simulink model "VCMGCM1962020b_v2"  (R2020b)
settings: Solver=FixedStepDiscrete  StartTime=0.0  StopTime=10.0  FixedStep=0.005  RelTol=1e-3  EnableMultiTasking=on
PreLoadFcn:
  | try, model_open; catch, disp('Error occurred while executing model pre-load callback: model_open.m'); disp('Please assure that the MATLAB working directory is set to the model directory before opening.'); end
InitFcn:
  | try, model_open; catch, end
undefined symbols (not defined in the file): Bridge, GCM, H, raptor_get_param_eval, raptor_get_safe_string, raptor_xcp_function
libraries: Blocks_lib x1165, Raptor_lib x665, simulink x62, VCM_lib x5
(part 1 of 23)
CloseFcn:
  | try, model_close; catch, end
settings Model: MotoHawkBuildVersion=501  MotoHawkBuildStats=struct('TotalFLASH',{0},'TotalEEPROM',{0},'TotalRAM',{0},'AppFLASH',{0},'AppEEPROM',{0},'AppRAM',{0},'HeapRAM',{0},'BuildSuccessCount',{170},'BuildErrorCount',{28})  MotoHawkModelSavedName=EVCM  MotoHawkModelGUID=11a0a5ad-fc23-4ada-98-f8-de-ae-e5-cd-40  MotoHawkModelOpenTime=2015 6 17 13 8 21.706  MotoHawkModelElapsedTime=81984019.981  MotoHawkBuildInfo=struct('model_name',{'EVCM'},'motohawk_version',{'2013a_sp0.336'},'motohawk_component_version',{'0.0.8'},'matlab_version',{'7.14.0'},'build_version',{'500'},'module_type',{'ECM-5554-112-0904-xD'},'layout_type',{'DEV'},'processor_family',{'MotoCoder'},'processor_type',{'MPC5554'},'toolchain_vendor',{'gcc-powerpc-eabispe'},'toolchain_version',{'4.6.0'},'component',{logical(0)},'archive_file',{''},'enable_build',{1},'fptype',{0},'flash_size',{2097152},'ee_size',{0},'ram_size',{65536},'decram_size',{0},'eri_table0_rev',{9},'max_eri_table_size',{65535},'use_debug_vardecs',{1},'use_info_vardecs',{1},'fgnd_base_period_ms',{5},'bgnd_base_period_ms',{100},'build_dir',{'C:\Users\Joe Morbitzer\Documents\Work - New Eagle\Projects\Base EV Supervisor Kit\EVCM_New\EVCM_Build'},'dll_name',{'EVCM_500'},'srz_name',{'EVCM_500'},'fgnd_stack_size',{3072},'fgnd_angle_stack_size',{0},'bgnd_stack_size',{2048},'idle_stack_size',{2048},'irq_stack_size',{1536},'heap_size',{4096},'heap_margin',{409},'install_dll_dir',{'C:\ECUFiles\TDBDLL'},'install_srz_dir',{'C:\ECUFiles\Programs\'},'app_int_stack_size',{2048},'shutdown_stack_size',{2048},'mingw_dir',{'C:\Program Files (x86)\Woodward\DevelopmentTools\Toolchains\GCC\win32-pe\4_4_0\'},'motohawk_dir',{'C:\Program Files (x86)\Woodward\MCS\MotoHawk\2013a_sp0.336'},'toolchain_dir',{'C:\Program Files (x86)\Woodward\DevelopmentTools\Toolchains\GCC\powerpc-eabispe\4_6_0'},'matlab_root',{'C:\Program Files\MATLAB\R2012a'},'model_guid',{'11a0a5ad-fc23-4ada-98-f8-de-ae-e5-cd-40'},'build_guid',{'47747e62-59be-442a-8d-e0-87-3b-e1-68-f2'},'token_guid',{'24876F82C12F5B448488EC225C14CAFD'})  MotoHawkBuildGUID=47747e62-59be-442a-8d-e0-87-3b-e1-68-f2  RegisteredStructs=struct('Name',{'FreezeFrame'},'Data',{struct('FltName',{0},'FltID',{0},'FltCount',{0},'RunTime',{0},'KeySw',{0})},'Enums',{{{'None','APP1InptHi','APP1InptLo','APP2InptHi','APP2InptLo','APPSnsCnflct','BPP1InptHi','BPP1InptLo','BPP2InptHi','BPP2InptLo','BPPSnsCnflct','DRVPVltHi','DRVPVltInptHi','DRVPVltInptLo','DRVPVltLo','EMTrqXChk','HVBCntrStck','HVBCurHi','HVBFlt','HVBNoTrnOn','HVBSOCLo','HVBTmpAvgHi1','HVBTmpAvgHi2','HVBTmpAvgHi3','HVBTmpAvgHi4','HVBTmpMxHi','HVBVltMnLo','HVBVltMxHi','HVSysFlt','KeySwVltHi','KeySwVltInptHi','KeySwVltInptLo','KeySwVltLo','MsgName1RxRateLo','MsgName2RxRateLo','PIMFlt','PIMNoTrnOn','PIMTmpHi1','PIMTmpHi2','PIMTmpHi3','PIMTmpHi4','Var11Inpt','Var21Inpt','VehSpdHi','XDRPVltHi','XDRPVltInptHi','XDRPVltInptLo','XDRPVltLo'},'',''}})  MotoHawkBuildDirectory=C:\Users\Joe Morbitzer\Documents\Work - New Eagle\Projects\Base EV Supervisor Kit\EVCM_New\EVCM_Build  RaptorUIDSize=4  Raptor_Target=GCM-1793-196-1503  Raptor_Calloc=NonVolatile (EEPROM)  RaptorFaultManager=OBD  RaptorBuildNum=67  Raptor_ecuaddr=253  Raptor_IsLiteMode=0  RaptorFaultManagerAddXYCounts=0  Creator=Joseph M. Morbitzer  LastModifiedBy=hratnam
settings ConfigSet: Description="This Simulink Configuration Set is preconfigured  for the MotoHawk target \"ECM-5554-112-0904-xD\"."
settings DataIOCC: LimitDataPoints=on  SaveFormat=Array  SignalLoggingSaveFormat=ModelDataLogs  ReturnWorkspaceOutputs=off
settings OptimizationCC: DefaultParameterBehavior=Inlined  UseSpecifiedMinMax=on  InlineInvariantSignals=on  EnhancedBackFolding=on  ExpressionDepthLimit=2147483647  InitFltsAndDblsToZero=on  NoFixptDivByZeroProtection=on  EfficientFloat2IntCast=on  LifeSpan=1  EfficientTunableParamExpr=on
settings DebuggingCC: ArtificialAlgebraicLoopMsg=none  InheritedTsInSrcMsg=none  TasksWithSamePriorityMsg=none  AllowSymbolicDim=off  StateNameClashWarn=warning  SFUnexpectedBacktrackingDiag=warning  SFNoUnconditionalDefaultTransitionDiag=warning  SFExecutionAtInitializationDiag=none  ArithmeticOperatorsInVariantConditions=warning
settings HardwareCC: ProdBitPerPointer=32  ProdBitPerSizeT=32  ProdBitPerPtrDiffT=32  ProdLargestAtomicFloat=None  ProdIntDivRoundTo=Undefined  ProdWordSize=32  ProdHWDeviceType=Infineon->TriCore  TargetIntDivRoundTo=Zero  TargetEndianess=LittleEndian  ProdEqTarget=off
settings ModelReferenceCC: UpdateModelReferenceTargets=AssumeUpToDate  CheckModelReferenceTargetMessage=none  ModelReferenceNumInstancesAllowed=Zero  PropagateSignalLabelsOutOfModel=off
settings SFSimCC: SimUseLocalCustomCode=off  MATLABDynamicMemAlloc=off  CustomCodeUndefinedFunction=UseInterfaceOnly
settings RTWCC: Description=Raptor (tm)  SystemTargetFile=raptor.tlc  GenCodeOnly=on  MakeCommand=raptor_make_rtw  TemplateMakefile=raptor.tmf  RTWUseLocalCustomCode=off
settings CodeAppCC: IgnoreCustomStorageClasses=off  MaxIdLength=100  CustomSymbolStrType=$N$R$M  CustomSymbolStrField=$H$N$M  StateflowObjectComments=on  InternalIdentifier=Classic
settings STFCustomTargetCC: GenerateSampleERTMain=on  ModelReferenceCompliant=off  ConcurrentExecutionCompliant=off  CombineOutputUpdateFcns=on  CombineSignalStateStructs=on  ERTCustomFileBanners=on  SupportComplex=off  SupportContinuousTime=off  SupportNonInlinedSFcns=off  RemoveResetFunc=on  MATLABClassNameForMDSCustomization=Simulink.SoftwareTarget.ERTCustomization  CPPClassGenCompliant=off  GRTInterface=off  SystemTargetFile=raptor.tlc
settings ERTTargetCC: MultiwordLength=2048  GenerateSampleERTMain=on  ModelReferenceCompliant=off  ParMdlRefBuildCompliant=off  CompOptLevelCompliant=off  ConcurrentExecutionCompliant=off  CombineSignalStateStructs=on  SupportComplex=off  ModelStepFunctionPrototypeControlCompliant=off  CPPClassGenCompliant=off  UseToolchainInfoCompliant=off  InlinedParameterPlacement=NonHierarchical  ERTCustomFileTemplate=example_file_process.tlc  SuppressUnreachableDefaultCases=off
settings ConfigComp: CovMetricSettings=dw  CovSaveCumulativeToWorkspaceVar=on  CovSaveSingleToWorkspaceVar=on  CovExternalEMLEnable=off

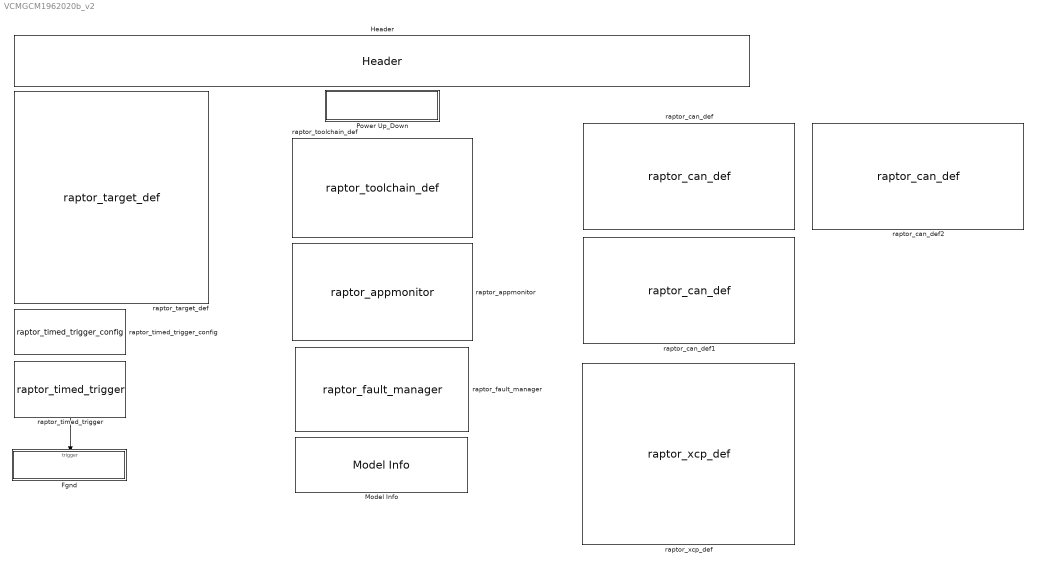
== system VCMGCM1962020b_v2 ==
  Fgnd : Subsystem  TreatAsAtomicUnit=on  mask{samptime=0.005}
      mask prompts: samptime "Sample Time (sec)"
      settings: RTWFcnNameOpts=Use subsystem name  RTWFileNameOpts=Use function name
      mask Display: disp(['Sample Time\n' num2str(samptime) ' sec']);
  Header : Blocks_lib/Header  width=Portrait  addtext=''
  Model Info : simulink/Model-Wide Utilities/Model Info  Frame=on  DisplayStringWithTags=|  HorizontalTextAlignment=Center  LeftAlignmentValue=0.5
      | Model Info
      | 
      | %<ModelVersion>
      | %<Description>
      | %<LastModifiedBy>
      | %<ModifiedComment>
  Power Up_Down : Subsystem  mask{group='Sensors | Voltage'}
  raptor_appmonitor : Raptor_lib/Application Monitoring/raptor_appmonitor  enabled=on  startupAction=Run  addStartupActionCal=off  minIdle=10  maxThread=70  calAccess=1  pctOverrunLimit=20  overrunAction=Count Occurrences  pauseOnReset=on  maxStackUsage=90  stackOverrunAction=Stop Application  addMaxStackCal=off  CANen=off
      settings: SourceProductName=Raptor
  raptor_can_def : Raptor_lib/CAN/raptor_can_def  canBus='CAN1'  resourceValues=CAN1|CAN2|CAN3|(None)  resource=CAN1  baudRateValues=125k|250k|500k|1000k  baudRate=250k  enable_baud_rate_config='RAPTOR MASK DEFAULT'  sim_func_name='RAPTOR MASK DEFAULT'  createButton=[]  txQueueSize=128  rxQueueSize=32
      settings: SourceProductName=Raptor
  raptor_can_def1 : Raptor_lib/CAN/raptor_can_def  canBus='CAN3'  resourceValues=CAN1|CAN2|CAN3|(None)  resource=CAN3  baudRateValues=125k|250k|500k|1000k  baudRate=500k  enable_baud_rate_config='RAPTOR MASK DEFAULT'  sim_func_name='RAPTOR MASK DEFAULT'  createButton=[]  txQueueSize=128  rxQueueSize=32
      settings: SourceProductName=Raptor
  raptor_can_def2 : Raptor_lib/CAN/raptor_can_def  canBus='CAN2'  resourceValues=CAN1|CAN2|CAN3|(None)  resource=CAN2  baudRateValues=125k|250k|500k|1000k  baudRate=250k  enable_baud_rate_config='RAPTOR MASK DEFAULT'  sim_func_name='RAPTOR MASK DEFAULT'  createButton=[]  txQueueSize=128  rxQueueSize=32
      settings: SourceProductName=Raptor
  raptor_fault_manager : Raptor_lib/Faults/raptor_fault_manager  button=0  managerTypeValues=Standard|OBD  managerType=OBD  cyclesToHeal=3  cyclesToClear=40  addXYCounts=0  calFaultMap=1  minFaultActions=2  minFaultTriggers=4  calAccessValues=4|3|2|1  calAccess=1  calFunction='Diagnostics'  initMap=struct()
      settings: SourceProductName=Raptor
  raptor_target_def : Raptor_lib/Configuration/raptor_target_def  targetValues=BCM-5646-48-1404|DISP-VC128-1901|DISP-VC320L-1402|DISP-VC320-1204|DISP-VC500-1904|DISP-VC700-2003|DISP-VC300R-2004|GCM-5634M-070-1459|GCM-5634M-070-1559|GCM-5634M-070-1562|ECM-1793-196-1503|GCM-1793-196-1503|GCM-5605B-048-1906|GCM-5607B-80-1901|GCM-5607B-80-1903|GCM-5607B-80-2001|RCM-5743R-080-2005|UAS-5743R-050-2006|GCM-5746R-048-1902|HCM-5604-36-1303|HCM-5604-36-1702  target=GCM-1793-196-1503  simpack=0  simulator=0  heap=2*1024  stack=2*1024  fgndStack=2*1024  bgndStack=2*1024  idleStack=1024  intStack=1536  sdStack=1024  appStack=1024  ecuaddr=253  uds_server_addr_ext=0  uds_server_addr=hex2dec('600')  uds_client_addr=hex2dec('650')  callocValues=Constant (FLASH)|NonVolatile (EEPROM)  calloc=NonVolatile (EEPROM)  compilerValues=HighTec v3.4.5.11  compiler=HighTec v3.4.5.11  setFileName=0  exeName=[raptor_get_safe_string(bdroot) '_']  addBuildNum=1  minVerChars=3  extraOutput=0  buildLocationValues=Raptor Default|Model Directory|User Defined  buildLocation=Raptor Default  exeLocation=''  a2lLocation=''  rpgLocation=''
      settings: SourceProductName=Raptor
  raptor_timed_trigger : Raptor_lib/Triggers/raptor_timed_trigger  triggerValues=Foreground|Foregroundx2|Foregroundx5|Foregroundx10|Foregroundx20|Background|Backgroundx2|Backgroundx5|Backgroundx10|Backgroundx20|Second|Minute  trigger=Foreground  inherited=0  alwaysEnabled=0  triggerPriority=0  triggerName=FGND_igkUo
      settings: SourceProductName=Raptor
  raptor_timed_trigger_config : Raptor_lib/Triggers/raptor_timed_trigger_config  triggerValues=Foreground|Background|Second|Minute  trigger=Foreground  period=5  CM2115newPeriod=5
      settings: SourceProductName=Raptor
  raptor_toolchain_def : Raptor_lib/Configuration/raptor_toolchain_def  matlabVer=9.9 (2020b)  raptorVer=2020b_2.2.13891  matCondition=Match Exactly  rapCondition=Match Exactly  matlabVerValues=9.9 (2020b)|9.8 (2020a)|9.7 (2019b)|9.6 (2019a)|9.5 (2018b)  matConditionValues=Match Exactly|Match or Newer|Match or Older  rapConditionValues=Match Exactly|Match or Newer|Match or Older
      settings: SourceProductName=Raptor
  raptor_xcp_def : Raptor_lib/Configuration/raptor_xcp_def  canBus='CAN1'  bcID=hex2dec('100')  bcID_TypeValues=Standard|Extended  bcID_Type=Standard  rxID=hex2dec('200')  rxID_TypeValues=Standard|Extended  rxID_Type=Standard  txID=hex2dec('300')  txID_TypeValues=Standard|Extended  txID_Type=Standard  daqRates=[5 10 100]  numODTs=80  genCANAPE=0  genVISION=0  securityValues=Standard|None|Custom User Defined  security=Standard  dllName=raptor_XCPSecurity.dll  accessValues=4|3|2|1  access=1
      settings: SourceProductName=Raptor
  wires:
  raptor_timed_trigger/1 -> Fgnd/Trigger

== system VCMGCM1962020b_v2/Fgnd ==
  f : TriggerPort  TriggerType=function-call  VariantControl=(inherit)
  Actuators : Subsystem
  Bus Creator : BusCreator  Inputs=5
  Bus Manager : Subsystem
  Control : Subsystem
  Diagnostics : Subsystem
  Header : Blocks_lib/Header  width=Portrait  addtext=''
  Sensors : Subsystem
  Virtual Sensors : Subsystem
  wires:
  Bus Manager/1(SBus) -> Sensors/1(Data)
  Bus Manager/2(VSBus) -> Virtual Sensors/1(Data)
  Bus Manager/3(CBus) -> Control/1(Data)
  Bus Manager/4(ABus) -> Actuators/1(Data)
  Bus Manager/5(DBus) -> Diagnostics/1(Data)
  Sensors/1(" Data") -> Bus Creator/1
  Virtual Sensors/1(" Data") -> Bus Creator/2
  Control/1(" Data") -> Bus Creator/3
  Actuators/1(" Data") -> Bus Creator/4
  Diagnostics/1(" Data") -> Bus Creator/5
  Bus Creator/1 -> Bus Manager/1(Data)

== system VCMGCM1962020b_v2/Power Up_Down ==
  Background : Subsystem
  raptor_timed_trigger : Raptor_lib/Triggers/raptor_timed_trigger  triggerValues=Foreground|Foregroundx2|Foregroundx5|Foregroundx10|Foregroundx20|Background|Backgroundx2|Backgroundx5|Backgroundx10|Backgroundx20|Second|Minute  trigger=Background  inherited=0  alwaysEnabled=1  triggerPriority=50  triggerName=BGND_kDJL0
      settings: SourceProductName=Raptor
  wires:
  raptor_timed_trigger/1 -> Background/Trigger

== system VCMGCM1962020b_v2/Fgnd/Actuators ==
  note: Old FMWS subsystem in case the j1939 implementation doesn't work
  Data : Inport
  Actuators : Subsystem
      settings: OpenFcn=open_system(gcb,'force')
  Bus Creator : BusCreator  Inputs=3
  CAN : Subsystem
  Command_G7 : Subsystem
      mask help:
      | Example of how to set up a CAN message transmit.
      | 1. Copy this block into the main model.
      | 2. Disable/break library link.
      | 3. Underneath, set up CAN Tx Message block.
      | 4. For each field, connect a CANTxField block from the CAN block to the bus creator; adjust parameters as necessary.
      mask init:
      | [msgnam, msgbus] = CANBlockInit('Tx');
      mask Display: disp(['CAN Tx: Message\n' msgnam '\n' msgbus]);
  FMWS : Subsystem  Commented=on  mask{nam='FMWS', bus='CAN1'}
      mask prompts: nam "Name"; bus "CAN Bus"
      mask Display: disp(['Forward Motion Warning System \n' nam '\n' bus]);
  FMWS_J1939 : Subsystem  mask{nam='FMWS', bus='CAN1'}
      mask prompts: nam "Name"; bus "CAN Bus"
      mask Display: disp(['Forward Motion Warning System \n' nam '\n' bus]);
  Header : Blocks_lib/Header  width=Portrait  addtext=''
  " Data" : Outport  VectorParamsAs1DForOutWhenUnconnected=off
  wires:
  Data/1 -> Command_G7/1(Data), FMWS_J1939/1(Data), CAN/1(Data), Actuators/1(Data)
  Bus Creator/1 -> " Data"/1  "Actuators"
  Actuators/1(Act) -> Bus Creator/1
  CAN/1(" CAN") -> Bus Creator/2
  FMWS_J1939/1(Act) -> Bus Creator/3

== system VCMGCM1962020b_v2/Fgnd/Bus Manager ==
  Data : Inport
  Bus Creator{,1..3} (4 alike) : BusCreator  Inputs=5
  Bus Selector : BusSelector  OutputSignals=Sensors
  Bus Selector1 : BusSelector  OutputSignals=VirtualSensors,Control,Actuators,Diagnostics
  Bus Selector2 : BusSelector  OutputSignals=Sensors,VirtualSensors
  Bus Selector3 : BusSelector  OutputSignals=Control,Actuators,Diagnostics
  Bus Selector4 : BusSelector  OutputSignals=Sensors,VirtualSensors,Control
  Bus Selector5 : BusSelector  OutputSignals=Actuators,Diagnostics
  Bus Selector6 : BusSelector  OutputSignals=Sensors,VirtualSensors,Control,Actuators
  Bus Selector7 : BusSelector  OutputSignals=Diagnostics
  Header : Blocks_lib/Header  width=Portrait  addtext=''
  Unit Delay : UnitDelay  SampleTime=-1  HasFrameUpgradeWarning=on
  SBus : Outport  VectorParamsAs1DForOutWhenUnconnected=off
  VSBus : Outport  Port=2  VectorParamsAs1DForOutWhenUnconnected=off
  CBus : Outport  Port=3  VectorParamsAs1DForOutWhenUnconnected=off
  ABus : Outport  Port=4  VectorParamsAs1DForOutWhenUnconnected=off
  DBus : Outport  Port=5  VectorParamsAs1DForOutWhenUnconnected=off
  wires:
  Bus Creator/1 -> SBus/1
  Bus Creator1/1 -> VSBus/1
  Bus Creator3/1 -> ABus/1
  Bus Creator2/1 -> CBus/1
  Bus Selector/1 -> Bus Creator/1  "<Sensors>"
  Bus Selector1/1 -> Bus Creator/2  "<VirtualSensors>"
  Bus Selector1/2 -> Bus Creator/3  "<Control>"
  Bus Selector1/3 -> Bus Creator/4  "<Actuators>"
  Bus Selector1/4 -> Bus Creator/5  "<Diagnostics>"
  Bus Selector4/1 -> Bus Creator2/1  "<Sensors>"
  Bus Selector4/2 -> Bus Creator2/2  "<VirtualSensors>"
  Bus Selector4/3 -> Bus Creator2/3  "<Control>"
  Bus Selector5/1 -> Bus Creator2/4  "<Actuators>"
  Bus Selector5/2 -> Bus Creator2/5  "<Diagnostics>"
  Bus Selector6/1 -> Bus Creator3/1  "<Sensors>"
  Bus Selector6/2 -> Bus Creator3/2  "<VirtualSensors>"
  Bus Selector6/3 -> Bus Creator3/3  "<Control>"
  Bus Selector6/4 -> Bus Creator3/4  "<Actuators>"
  Bus Selector7/1 -> Bus Creator3/5  "<Diagnostics>"
  Data/1 -> Bus Selector/1, Bus Selector2/1, Bus Selector4/1, Bus Selector6/1, DBus/1, Unit Delay/1
  Unit Delay/1 -> Bus Selector1/1, Bus Selector3/1, Bus Selector5/1, Bus Selector7/1
  Bus Selector2/1 -> Bus Creator1/1  "<Sensors>"
  Bus Selector2/2 -> Bus Creator1/2  "<VirtualSensors>"
  Bus Selector3/1 -> Bus Creator1/3  "<Control>"
  Bus Selector3/2 -> Bus Creator1/4  "<Actuators>"
  Bus Selector3/3 -> Bus Creator1/5  "<Diagnostics>"

== system VCMGCM1962020b_v2/Fgnd/Control ==
  Data : Inport
  Battery : Subsystem
  Bus Creator : BusCreator  Inputs=8
  Charger : Subsystem
  DC/DC Converter : Subsystem
  Drive Inverter : Subsystem  mask{group='Control | Drive Inverter'}
  EPAS : Subsystem
  Header : Blocks_lib/Header  width=Portrait  addtext=''
  Modes : Subsystem  mask{group='Control | Modes'}
  Other : Subsystem
  PDU : Subsystem
  " Data" : Outport  VectorParamsAs1DForOutWhenUnconnected=off
  wires:
  Modes/1(Ctrl) -> Bus Creator/1
  Battery/1(Ctrl) -> Bus Creator/2
  PDU/1(Ctrl) -> Bus Creator/3
  Charger/1(Ctrl) -> Bus Creator/4
  DC/DC Converter/1(Ctrl) -> Bus Creator/5
  Drive Inverter/1(Ctrl) -> Bus Creator/6
  Other/1(Ctrl) -> Bus Creator/7
  Bus Creator/1 -> " Data"/1  "Control"
  Data/1 -> Modes/1(Data), PDU/1(Data), DC/DC Converter/1(Data), Drive Inverter/1(Data), EPAS/1(Data), Other/1(Data), Charger/1(Data), Battery/1(Data)
  EPAS/1(Ctrl) -> Bus Creator/8

== system VCMGCM1962020b_v2/Fgnd/Diagnostics ==
  Data : Inport
  Diagnostics : Subsystem
  Fault Statuses : Subsystem  mask{group='Diagnostics | Fault Statuses'}
  Ground : Ground
  Header : Blocks_lib/Header  width=Portrait  addtext=''
  " Data" : Outport  VectorParamsAs1DForOutWhenUnconnected=off
  wires:
  Ground/1 -> " Data"/1  "Diagnostics"
  Data/1 -> Diagnostics/1(Data), Fault Statuses/1(Data)

== system VCMGCM1962020b_v2/Fgnd/Sensors ==
  Data : Inport
  Bus Creator : BusCreator  Inputs=2
  CAN : Subsystem
      settings: OpenFcn=open_system(gcb,'force')
  Header : Blocks_lib/Header  width=Portrait  addtext=''
  Sensors : Subsystem
      settings: OpenFcn=open_system(gcb,'force')
  " Data" : Outport  VectorParamsAs1DForOutWhenUnconnected=off
  wires:
  Sensors/1(Sns) -> Bus Creator/1
  CAN/1(CAN) -> Bus Creator/2
  Bus Creator/1 -> " Data"/1  "Sensors"
  Data/1 -> Sensors/1(Data), CAN/1(Data)

== system VCMGCM1962020b_v2/Fgnd/Virtual Sensors ==
  note: Note:
      | These subsystems provide a common interface
      | to the rest of the model for the core data whose
      | source is application-dependent and/or may
      | need adjustment to match the model convention.
  Data : Inport
  Battery : Subsystem
  Bus Creator : BusCreator  Inputs=8
  Charger : Subsystem
  DC/DC Converter : Subsystem
  Drive Inverter : Subsystem
  Driver Inputs : Subsystem
  Header : Blocks_lib/Header  width=Portrait  addtext=''
  Other : Subsystem
  PDU : Subsystem
  Vehicle : Subsystem
  " Data" : Outport  VectorParamsAs1DForOutWhenUnconnected=off
  wires:
  Bus Creator/1 -> " Data"/1  "VirtualSensors"
  Driver Inputs/1(" Data") -> Bus Creator/1
  Battery/1(" Data") -> Bus Creator/2
  PDU/1(" Data") -> Bus Creator/3
  Charger/1(" Data") -> Bus Creator/4
  DC/DC Converter/1(" Data") -> Bus Creator/5
  Drive Inverter/1(" Data") -> Bus Creator/6
  Vehicle/1(" Data") -> Bus Creator/7
  Data/1 -> Driver Inputs/1(Data), PDU/1(Data), Charger/1(Data), DC/DC Converter/1(Data), Drive Inverter/1(Data), Other/1(Data), Vehicle/1(Data), Battery/1(Data)
  Other/1(" Data") -> Bus Creator/8

== system VCMGCM1962020b_v2/Power Up_Down/Background ==
  note: Notes :
      | - Calling the shutdown task stops the foreground tasks. However, background tasks continue, so the reading of key switch must be in this subsystem to allow the module
      | to resume operation (by calling the startup task) if keyswitch is turned back on before the module actually turns off.
      | - The Startup Event is automatically called when the module is powered on after being completely off. The FgndTasksStopped data store prevents the Startup Event from being called twice in this scenario.
  f : TriggerPort  TriggerType=function-call  VariantControl=(inherit)  ZeroCross=off
  Debounce : Subsystem
  Logical Operator1 : Logic  Operator=OR  OutDataTypeStr=boolean
  Logical Operator2 : Logic  Operator=OR  Inputs=3  OutDataTypeStr=boolean
  Raise Shutdown Event : Subsystem  TreatAsAtomicUnit=on
  Raise Startup Event : Subsystem  TreatAsAtomicUnit=on
  Store EEPROM : Subsystem  TreatAsAtomicUnit=on
  Unit Delay : UnitDelay  SampleTime=-1  HasFrameUpgradeWarning=on
  Unit Delay1 : UnitDelay  SampleTime=-1  HasFrameUpgradeWarning=on
  raptor_data_def : Raptor_lib/Data Storage/raptor_data_def  dataName='Wake_Bgnd'  initValue=0  dataType=boolean  storage=Volatile (RAM)  calVisible=on  calType=Measurement  calDispType=Number  calEnum={'False', 'True'}  calGain=1.0  calOffset=0  calMin=-Inf  calMax=Inf  calFormat='-1'  calUnit='Bool'  calHelp='Wake reading from background task'  calAccess=1  calFunction=group  calDispHeaders=off  calColHeaders={'Col1' 'Col2' 'Col3'}  calRowHeaders={'Row1' 'Row2' 'Row3'}
      settings: SourceProductName=Raptor
  raptor_data_def1 : Raptor_lib/Data Storage/raptor_data_def  dataName='KeepModuleOn'  initValue=0  dataType=boolean  storage=Volatile (RAM)  calVisible=on  calType=Measurement  calDispType=Number  calEnum={'False', 'True'}  calGain=1.0  calOffset=0  calMin=-Inf  calMax=Inf  calFormat='-1'  calUnit='Bool'  calHelp='Module to be kept on'  calAccess=1  calFunction=group  calDispHeaders=off  calColHeaders={'Col1' 'Col2' 'Col3'}  calRowHeaders={'Row1' 'Row2' 'Row3'}
      settings: SourceProductName=Raptor
  raptor_data_read : Raptor_lib/Data Storage/raptor_data_read  dataName='FgndTasksStopped'  dataShape=Scalar  idxSource=Input  idxRow=1  idxCol=1
      settings: SourceProductName=Raptor
  raptor_data_read1 : Raptor_lib/Data Storage/raptor_data_read  dataName='KeepModuleOn'  dataShape=Scalar  idxSource=Input  idxRow=1  idxCol=1
      settings: SourceProductName=Raptor
  raptor_data_write : Raptor_lib/Data Storage/raptor_data_write  dataName='Wake_Bgnd'  dataShape=Scalar  idxSource=Input Port  idxRow=1  idxCol=1
      settings: SourceProductName=Raptor
  raptor_digital_in : Raptor_lib/Input & Output/raptor_digital_in  resourceValues=(None)|WAKE_INPUT1|INPUT33|INPUT34|INPUT35|INPUT36|INPUT37|INPUT38|INPUT39|INPUT40  resource=WAKE_INPUT1  pullUDValues=2.9k PD  pullUD=2.9k PD  upperThres=1.980  lowerThres=1.320
      settings: SourceProductName=Raptor
  raptor_digital_out : Raptor_lib/Input & Output/raptor_digital_out  resourceValues=OUTPUT9|OUTPUT21|OUTPUT22|OUTPUT23|OUTPUT24|(None)|OUTPUT1|OUTPUT2|OUTPUT3|OUTPUT4|OUTPUT5|OUTPUT6|OUTPUT7|OUTPUT8|OUTPUT10|OUTPUT11|OUTPUT25|OUTPUT26|OUTPUT27|OUTPUT28|OUTPUT29|OUTPUT30|OUTPUT31|OUTPUT32|OUTPUT33|OUTPUT34|OUTPUT35|OUTPUT36|OUTPUT37|OUTPUT38|OUTPUT39|OUTPUT40|OUTPUT41|OUTPUT42|OUTPUT43|OUTPUT44|OUTPUT45|OUTPUT46|OUTPUT47|OUTPUT48|POWER_HOLD  resource=POWER_HOLD  driverTypeValues=(None)  driverType=(None)
      settings: SourceProductName=Raptor
  raptor_sfun_nv_status : Raptor_lib/Data Storage/raptor_sfun_nv_status  showStatus=Store In Progess
      settings: SourceProductName=Raptor
  wires:
  raptor_data_read/1 -> Raise Startup Event/Enable
  Debounce/1(Out) -> Logical Operator1/1, raptor_data_write/1
  raptor_data_read1/1 -> Logical Operator1/2
  raptor_digital_in/1 -> Debounce/1(In)
  Logical Operator2/1 -> raptor_digital_out/1
  Unit Delay/1 -> Store EEPROM/Trigger, Unit Delay1/1
  Logical Operator1/1 -> Logical Operator2/2, Raise Startup Event/Trigger, Raise Shutdown Event/Trigger, Unit Delay/1
  Unit Delay1/1 -> Logical Operator2/3
  raptor_sfun_nv_status/1 -> Logical Operator2/1

== system VCMGCM1962020b_v2/Fgnd/Actuators/Actuators ==
  Data : Inport
  Bus Creator : BusCreator  Inputs=2
  Header : Blocks_lib/Header  width=Portrait  addtext=''
  Other : Subsystem
      settings: OpenFcn=open_system(gcb,'force')
  PDU : Subsystem
      mask Display: disp('PDU: New Eagle');
  Act : Outport  VectorParamsAs1DForOutWhenUnconnected=off
  wires:
  Bus Creator/1 -> Act/1  "Actuators"
  PDU/1(Act) -> Bus Creator/1
  Other/1(Act) -> Bus Creator/2
  Data/1 -> Other/1(Data), PDU/1(Data)

== system VCMGCM1962020b_v2/Fgnd/Actuators/CAN ==
  Data : Inport
  Battery : Subsystem  mask{nam='Chgr', bus='CAN1'}
      mask prompts: nam "Name"; bus "CAN Bus"
      mask Display: disp(['Battery: Romeo\n' nam '\n' bus]);
  Body Control : Subsystem  mask{nam='BCM', bus='CAN1'}
      mask prompts: nam "Name"; bus "CAN Bus"
      mask Display: disp(['Body Control Module \n' nam '\n' bus]);
  Bus Creator : BusCreator  Inputs=8
  CCS Interface : Subsystem  Commented=on  mask{nam='CCS', bus='CAN1'}
      mask prompts: nam "Name"; bus "CAN Bus"
      mask Display: disp(['CCS Interface: IoTecha M2iEV\n' nam '\n' bus]);
  Charger : Subsystem  mask{nam='Chgr', bus='CAN1'}
      mask prompts: nam "Name"; bus "CAN Bus"
      mask Display: disp(['On-Board Charger: Dilong 3.3k\n' nam '\n' bus]);
  DC/DC Converter : Subsystem  Commented=on  mask{nam='DCDC', bus='CAN1'}
      mask prompts: nam "Name"; bus "CAN Bus"
      mask Display: disp(['DC/DC Converter: Bel Power DNC\n' nam '\n' bus]);
  DC/DC Converter1 : Subsystem  mask{nam='DCDC', bus='CAN1'}
      mask prompts: nam "Name"; bus "CAN Bus"
      mask Display: disp(['DC/DC Converter: Dilong 0-16V\n' nam '\n' bus]);
  Display : Subsystem  mask{nam='Display', bus='CAN1'}
      mask prompts: nam "Name"; bus "CAN Bus"
      mask Display: disp(['Driver Display\n' nam '\n' bus]);
  Drive Inverter : Subsystem  mask{nam='DrvInvtr', bus='CAN3'}
      mask prompts: nam "Name"; bus "CAN Bus"
      mask Display: disp(['Inverter: Saietta\n' nam '\n' bus]);
  Header : Blocks_lib/Header  width=Portrait  addtext=''
  Other : Subsystem  Commented=on
      settings: OpenFcn=open_system(gcb,'force')
  " CAN" : Outport  VectorParamsAs1DForOutWhenUnconnected=off
  wires:
  CCS Interface/1(Act) -> Bus Creator/2
  Bus Creator/1 -> " CAN"/1  "CAN"
  Data/1 -> CCS Interface/1(Data), Battery/1(Data), Charger/1(Data), DC/DC Converter1/1(Data), Drive Inverter/1(Data), Display/1(Data), Body Control/1(Data), Other/1(Data)
  Charger/1(Act) -> Bus Creator/3
  DC/DC Converter1/1(Act) -> Bus Creator/4
  Drive Inverter/1(Act) -> Bus Creator/5
  Other/1(CAN) -> Bus Creator/6
  Battery/1(Act) -> Bus Creator/1
  Body Control/1(Act) -> Bus Creator/7
  Display/1(Act) -> Bus Creator/8

== system VCMGCM1962020b_v2/Fgnd/Actuators/Command_G7 ==
  note: For some reason the bus doesn't initalize with signals when inside the subsystem. Tried updating it multiple times
  Data : Inport
  Bus Selector : BusSelector  OutputSignals=Control.Mode.StartStop.ModWake [Bool]
  Bus Selector1 : BusSelector  OutputSignals=Control.EPASCmmd [Bool]
  CANTxMsgEnbl : Blocks_lib/CANTxMsgEnbl  custom=off  custom_nam='---'  msgnam=Command_G7
  Header : Blocks_lib/Header  width=Portrait  addtext=''
  MsgTx : Subsystem
  wires:
  CANTxMsgEnbl/1 -> MsgTx/Enable
  Data/1 -> Bus Selector1/1, Bus Selector/1
  Bus Selector/1 -> CANTxMsgEnbl/1  "<ModWake [Bool]>"
  Bus Selector1/1 -> MsgTx/1(Data)  "<EPASCmmd [Bool]>"

== system VCMGCM1962020b_v2/Fgnd/Actuators/FMWS ==
  Data : Inport
  Ground : Ground
  Header : Blocks_lib/Header  width=Portrait  addtext=''
  MCU_130h : Subsystem
      mask help:
      | Example of how to set up a CAN message transmit.
      | 1. Copy this block into the main model.
      | 2. Disable/break library link.
      | 3. Underneath, set up CAN Tx Message block.
      | 4. For each field, connect a CANTxField block from the CAN block to the bus creator; adjust parameters as necessary.
      mask init:
      | [msgnam, msgbus] = CANBlockInit('Tx');
      mask Display: disp(['CAN Tx: Message\n' msgnam '\n' msgbus]);
  MCU_131h : Subsystem
      mask help:
      | Example of how to set up a CAN message transmit.
      | 1. Copy this block into the main model.
      | 2. Disable/break library link.
      | 3. Underneath, set up CAN Tx Message block.
      | 4. For each field, connect a CANTxField block from the CAN block to the bus creator; adjust parameters as necessary.
      mask init:
      | [msgnam, msgbus] = CANBlockInit('Tx');
      mask Display: disp(['CAN Tx: Message\n' msgnam '\n' msgbus]);
  Act : Outport  VectorParamsAs1DForOutWhenUnconnected=off
  wires:
  Ground/1 -> Act/1  "FMWS"
  Data/1 -> MCU_130h/1(Data), MCU_131h/1(Data)

== system VCMGCM1962020b_v2/Fgnd/Actuators/FMWS_J1939 ==
  Data : Inport
  CCVS : Subsystem
      mask help:
      | Example of how to set up a CAN message transmit.
      | 1. Copy this block into the main model.
      | 2. Disable/break library link.
      | 3. Underneath, set up CAN Tx Message block.
      | 4. For each field, connect a CANTxField block from the CAN block to the bus creator; adjust parameters as necessary.
      mask init:
      | [msgnam, msgbus] = CANBlockInit('Tx');
      mask Display: disp(['CAN Tx: Message\n' msgnam '\n' msgbus]);
  ETC2 : Subsystem
      mask help:
      | Example of how to set up a CAN message transmit.
      | 1. Copy this block into the main model.
      | 2. Disable/break library link.
      | 3. Underneath, set up CAN Tx Message block.
      | 4. For each field, connect a CANTxField block from the CAN block to the bus creator; adjust parameters as necessary.
      mask init:
      | [msgnam, msgbus] = CANBlockInit('Tx');
      mask Display: disp(['CAN Tx: Message\n' msgnam '\n' msgbus]);
  Ground : Ground
  Header : Blocks_lib/Header  width=Portrait  addtext=''
  Act : Outport  VectorParamsAs1DForOutWhenUnconnected=off
  wires:
  Data/1 -> ETC2/1(Data), CCVS/1(Data)
  Ground/1 -> Act/1  "FMWS"

== system VCMGCM1962020b_v2/Fgnd/Control/Battery ==
  Data : Inport
  Bus Creator : BusCreator  Inputs=2
  Bus Selector : BusSelector  OutputSignals=VirtualSensors.Batt.MaxBattVoltsVld [bool],VirtualSensors.Batt.MaxBattVolts [V]
  Header : Blocks_lib/Header  width=Portrait  addtext=''
  Min : MinMax  Inputs=2
  Multiport Switch : MultiPortSwitch  DataPortOrder=Zero-based contiguous  Inputs=2  zeroidx=on
  raptor_adjustment : Raptor_lib/Data Storage/raptor_adjustment  paramName='BattIsoTestEnbl'  nameSource=Parameter  initValue=true  dataType=double  storage=Calibration  calDispType=Number  calEnum={'False', 'True'}  calGain=1.0  calOffset=0.0  calMax=inf  calMin=-inf  calFormat='-1'  calUnit='bool'  calHelp='Enable Passive Battery Isolation test'  calAccess=1  calFunction='Control | Battery'  calDispHeaders=off  calColHeaders={'Col1' 'Col2' 'Col3'}  calRowHeaders={'Row1' 'Row2' 'Row3'}
      settings: SourceProductName=Raptor
  raptor_adjustment1 : Raptor_lib/Data Storage/raptor_adjustment  paramName='BattMaxAllVoltage'  nameSource=Parameter  initValue=100  dataType=double  storage=Calibration  calDispType=Number  calEnum={'False', 'True'}  calGain=1.0  calOffset=0.0  calMax=inf  calMin=-inf  calFormat='-1'  calUnit='V'  calHelp='Calibration battery Voltage Limit (for charging)'  calAccess=1  calFunction='Control | Battery'  calDispHeaders=off  calColHeaders={'Col1' 'Col2' 'Col3'}  calRowHeaders={'Row1' 'Row2' 'Row3'}
      settings: SourceProductName=Raptor
  Ctrl : Outport  VectorParamsAs1DForOutWhenUnconnected=off
  wires:
  Bus Creator/1 -> Ctrl/1  "Batt"
  raptor_adjustment/1 -> Bus Creator/1  "BattIsoTestEnbl [Bool]"
  Data/1 -> Bus Selector/1
  Bus Selector/1 -> Multiport Switch/1  "<MaxBattVoltsVld [bool]>"
  raptor_adjustment1/1 -> Multiport Switch/2, Min/1  "BattIsoTestEnbl [Bool]"
  Bus Selector/2 -> Min/2  "<MaxBattVolts [V]>"
  Min/1 -> Multiport Switch/3
  Multiport Switch/1 -> Bus Creator/2  "MaxVoltAllow"

== system VCMGCM1962020b_v2/Fgnd/Control/Charger ==
  note: EVSUP
  Data : Inport
  Add : Sum  InputSameDT=on  OutDataTypeStr=Inherit: Same as first input
  Bus Creator : BusCreator  Inputs=6
  Bus Selector : BusSelector  OutputSignals=VirtualSensors.Chgr.OnBoard.OnBoardChgr [Bool],Control.Mode.StartStop.ChgMode [Bool]
  Bus Selector1 : BusSelector  OutputSignals=VirtualSensors.Chgr.OnBoard.OnBoardChgrEVSEACCurLim [A]
  Bus Selector2 : BusSelector  OutputSignals=VirtualSensors.Batt.BattCCL [A],VirtualSensors.PDU.HVAccCur [A]
  Bus Selector3 : BusSelector  Commented=on  OutputSignals=VirtualSensors.Chgr.OffBoard.OffBoardChgrEVSEDCCurLim [A]
  Bus Selector4 : BusSelector  Commented=on  OutputSignals=Control.Batt.MaxVoltAllow
  Bus Selector5 : BusSelector  OutputSignals=VirtualSensors.Batt.BattChgComplete [Bool]
  Ground : Ground
  Header : Blocks_lib/Header  width=Portrait  addtext=''
  Logical Operator : Logic  Inputs=3  AllPortsSameDT=off  OutDataTypeStr=boolean
  MinMax : MinMax  Inputs=2
  MinMax1 : MinMax  Inputs=2
  MinMax2 : MinMax  Commented=on  Inputs=3
  NOT : Logic  Operator=NOT  AllPortsSameDT=off  OutDataTypeStr=boolean
  Switch : Switch  Criteria=u2 > Threshold
  Zero-Order Hold : ZeroOrderHold  SampleTime=-1
  Zero-Order Hold1 : ZeroOrderHold  SampleTime=-1
  raptor_adjustment : Raptor_lib/Data Storage/raptor_adjustment  paramName='OnBoardChgrEnblReqEnbl'  nameSource=Parameter  initValue=0  dataType=boolean  storage=Calibration  calDispType=Number  calEnum={'False', 'True'}  calGain=1  calOffset=0  calMax=inf  calMin=-inf  calFormat=''  calUnit='Bool'  calHelp='On-board charger enable request enable'  calAccess=1  calFunction='Control | Charger'  calDispHeaders=off  calColHeaders={'Col1' 'Col2' 'Col3'}  calRowHeaders={'Row1' 'Row2' 'Row3'}
      settings: SourceProductName=Raptor
  raptor_adjustment1 : Raptor_lib/Data Storage/raptor_adjustment  paramName='ChgrDCVoltSetpt'  nameSource=Parameter  initValue=0  dataType=double  storage=Calibration  calDispType=Number  calEnum={'Disabled', 'Enabled'}  calGain=1  calOffset=0  calMax=inf  calMin=-inf  calFormat=''  calUnit='V'  calHelp='Charger DC voltage setpoint'  calAccess=1  calFunction='Control | Charger'  calDispHeaders=off  calColHeaders={'Col1' 'Col2' 'Col3'}  calRowHeaders={'Row1' 'Row2' 'Row3'}
      settings: SourceProductName=Raptor
  raptor_adjustment2 : Raptor_lib/Data Storage/raptor_adjustment  paramName='OnBoardChgrACCurLim'  nameSource=Parameter  initValue=0  dataType=double  storage=Calibration  calDispType=Number  calEnum={'Disabled', 'Enabled'}  calGain=1  calOffset=0  calMax=inf  calMin=-inf  calFormat=''  calUnit='A'  calHelp='On-board charger AC current limit'  calAccess=1  calFunction='Control | Charger'  calDispHeaders=off  calColHeaders={'Col1' 'Col2' 'Col3'}  calRowHeaders={'Row1' 'Row2' 'Row3'}
      settings: SourceProductName=Raptor
  raptor_adjustment3 : Raptor_lib/Data Storage/raptor_adjustment  paramName='OnBoardChgrDCCurLim'  nameSource=Parameter  initValue=0  dataType=double  storage=Calibration  calDispType=Number  calEnum={'Disabled', 'Enabled'}  calGain=1  calOffset=0  calMax=inf  calMin=-inf  calFormat=''  calUnit='A'  calHelp='On-board charger DC current limit'  calAccess=1  calFunction='Control | Charger'  calDispHeaders=off  calColHeaders={'Col1' 'Col2' 'Col3'}  calRowHeaders={'Row1' 'Row2' 'Row3'}
      settings: SourceProductName=Raptor
  raptor_adjustment4 : Raptor_lib/Data Storage/raptor_adjustment  Commented=on  paramName='OffBoardChgrDCCurLim'  nameSource=Parameter  initValue=0  dataType=double  storage=Calibration  calDispType=Number  calEnum={'Disabled', 'Enabled'}  calGain=1  calOffset=0  calMax=inf  calMin=-inf  calFormat=''  calUnit='A'  calHelp='Off-board charger DC current limit'  calAccess=1  calFunction='Control | Charger'  calDispHeaders=off  calColHeaders={'Col1' 'Col2' 'Col3'}  calRowHeaders={'Row1' 'Row2' 'Row3'}
      settings: SourceProductName=Raptor
  raptor_adjustment5 : Raptor_lib/Data Storage/raptor_adjustment  paramName='OnBoardChgrDCCurLimLVChrgOnly'  nameSource=Parameter  initValue=3  dataType=double  storage=Calibration  calDispType=Number  calEnum={'Disabled', 'Enabled'}  calGain=1  calOffset=0  calMax=inf  calMin=-inf  calFormat=''  calUnit='A'  calHelp='On-board charger DC current limit when only charging LV battery system'  calAccess=1  calFunction='Control | Charger'  calDispHeaders=off  calColHeaders={'Col1' 'Col2' 'Col3'}  calRowHeaders={'Row1' 'Row2' 'Row3'}
      settings: SourceProductName=Raptor
  Ctrl : Outport  VectorParamsAs1DForOutWhenUnconnected=off
  wires:
  Bus Selector/1 -> Logical Operator/2  "<OnBoardChgr [Bool]>"
  Bus Creator/1 -> Ctrl/1  "Chgr"
  raptor_adjustment1/1 -> Bus Creator/2  "ChgrDCVoltSetpt [V]"
  Logical Operator/1 -> Bus Creator/1  "OnBoardChgrEnblReq [Bool]"
  raptor_adjustment/1 -> Logical Operator/1
  Bus Selector/2 -> Logical Operator/3  "<ChgMode [Bool]>"
  MinMax/1 -> Bus Creator/3  "OnBoardChgrACCurLim [A]"
  raptor_adjustment2/1 -> MinMax/2
  Bus Selector1/1 -> MinMax/1  "<OnBoardChgrEVSEACCurLim [A]>"
  MinMax1/1 -> Bus Creator/4  "OnBoardChgrDCCurLim [A]"
  Add/1 -> Switch/1
  raptor_adjustment3/1 -> MinMax1/2
  Bus Selector2/1 -> Add/1  "<BattCCL [A]>"
  Zero-Order Hold/1 -> Bus Creator/5  "OffBoardChgrDCCurLim [A]"
  Bus Selector3/1 -> MinMax2/2  "<OffBoardChgrEVSEDCCurLim [A]>"
  raptor_adjustment4/1 -> MinMax2/3
  Data/1 -> Bus Selector5/1, Bus Selector2/1, Bus Selector1/1, Bus Selector/1
  Bus Selector2/2 -> Add/2  "<HVAccCur [A]>"
  Zero-Order Hold1/1 -> Bus Creator/6  "MaxVoltAllowed [V]"
  Ground/1 -> Zero-Order Hold1/1, Zero-Order Hold/1
  Bus Selector5/1 -> NOT/1  "<BattChgComplete [Bool]>"
  NOT/1 -> Switch/2
  raptor_adjustment5/1 -> Switch/3
  Switch/1 -> MinMax1/1

== system VCMGCM1962020b_v2/Fgnd/Control/DC//DC Converter ==
  Data : Inport
  Bus Creator : BusCreator  Inputs=3
  Bus Selector : BusSelector  OutputSignals=Control.Mode.StartStop.ChgMode [Bool],Control.Mode.StartStop.RunMode [Bool]
  Header : Blocks_lib/Header  width=Portrait  addtext=''
  Logical Operator : Logic  Operator=OR  OutDataTypeStr=boolean
  Logical Operator1 : Logic  OutDataTypeStr=boolean
  raptor_adjustment : Raptor_lib/Data Storage/raptor_adjustment  paramName='DCDCEnblReqEnbl'  nameSource=Parameter  initValue=0  dataType=boolean  storage=Calibration  calDispType=Number  calEnum={'False', 'True'}  calGain=1  calOffset=0  calMax=inf  calMin=-inf  calFormat=''  calUnit='Bool'  calHelp='DC/DC converter enable request enable'  calAccess=1  calFunction='Control | DCDC'  calDispHeaders=off  calColHeaders={'Col1' 'Col2' 'Col3'}  calRowHeaders={'Row1' 'Row2' 'Row3'}
      settings: SourceProductName=Raptor
  raptor_adjustment1 : Raptor_lib/Data Storage/raptor_adjustment  paramName='DCDCOutptVoltSetpt'  nameSource=Parameter  initValue=0  dataType=double  storage=Calibration  calDispType=Number  calEnum={'Disabled', 'Enabled'}  calGain=1  calOffset=0  calMax=inf  calMin=-inf  calFormat=''  calUnit='V'  calHelp='DC/DC converter output voltage setpoint'  calAccess=1  calFunction='Control | DCDC'  calDispHeaders=off  calColHeaders={'Col1' 'Col2' 'Col3'}  calRowHeaders={'Row1' 'Row2' 'Row3'}
      settings: SourceProductName=Raptor
  raptor_adjustment2 : Raptor_lib/Data Storage/raptor_adjustment  paramName='DCDCOutptCurLim'  nameSource=Parameter  initValue=0  dataType=double  storage=Calibration  calDispType=Number  calEnum={'Disabled', 'Enabled'}  calGain=1  calOffset=0  calMax=inf  calMin=-inf  calFormat=''  calUnit='A'  calHelp='DC/DC converter output current limit'  calAccess=1  calFunction='Control | DCDC'  calDispHeaders=off  calColHeaders={'Col1' 'Col2' 'Col3'}  calRowHeaders={'Row1' 'Row2' 'Row3'}
      settings: SourceProductName=Raptor
  Ctrl : Outport  VectorParamsAs1DForOutWhenUnconnected=off
  wires:
  raptor_adjustment1/1 -> Bus Creator/2  "DCDCOutptVoltSetpt [V]"
  Bus Creator/1 -> Ctrl/1  "DCDC"
  Logical Operator1/1 -> Bus Creator/1  "DCDCEnblReq [Bool]"
  raptor_adjustment2/1 -> Bus Creator/3  "DCDCOutptCurLim [A]"
  Bus Selector/1 -> Logical Operator/1  "<ChgMode [Bool]>"
  Bus Selector/2 -> Logical Operator/2  "<RunMode [Bool]>"
  Logical Operator/1 -> Logical Operator1/2
  raptor_adjustment/1 -> Logical Operator1/1
  Data/1 -> Bus Selector/1

== system VCMGCM1962020b_v2/Fgnd/Control/Drive Inverter ==
  Data : Inport
  Bus Creator : BusCreator  Inputs=2
  Header : Blocks_lib/Header  width=Portrait  addtext=''
  Inverter Enable Request : Subsystem
  Motor Torque Request : Subsystem
  Ctrl : Outport  VectorParamsAs1DForOutWhenUnconnected=off
  wires:
  Bus Creator/1 -> Ctrl/1  "DrvInvtr"
  Motor Torque Request/1(MtrTrqReq) -> Bus Creator/2
  Inverter Enable Request/1(Bool) -> Bus Creator/1, Motor Torque Request/2(EnblReq)  "DrvInvtrEnblReq [Bool]"
  Data/1 -> Motor Torque Request/1(Data), Inverter Enable Request/1(Data)

== system VCMGCM1962020b_v2/Fgnd/Control/EPAS ==
  Data : Inport
  Bus Selector : BusSelector  OutputSignals=Sensors.Sensors.Volt.Wake [Bool]
  Header : Blocks_lib/Header  width=Portrait  addtext=''
  Zero-Order Hold : ZeroOrderHold  SampleTime=-1
  Ctrl : Outport  VectorParamsAs1DForOutWhenUnconnected=off
  wires:
  Data/1 -> Bus Selector/1
  Bus Selector/1 -> Zero-Order Hold/1  "<Wake [Bool]>"
  Zero-Order Hold/1 -> Ctrl/1  "EPASCmmd [Bool]"

== system VCMGCM1962020b_v2/Fgnd/Control/Modes ==
  Data : Inport
  Bus Creator : BusCreator  Inputs=4
  Header : Blocks_lib/Header  width=Portrait  addtext=''
  PRND Mode : Subsystem
  Startup & Shutdown : Subsystem
  Ctrl : Outport  VectorParamsAs1DForOutWhenUnconnected=off
  wires:
  Bus Creator/1 -> Ctrl/1  "Mode"
  PRND Mode/1(enum) -> Bus Creator/2  "PRNDMode [enum]"
  Startup & Shutdown/1(Ctrl) -> Bus Creator/1
  Data/1 -> PRND Mode/1(Data), Startup & Shutdown/1(Data)
  PRND Mode/2(enum1) -> Bus Creator/3  "PRNDMode_Act [enum]"
  PRND Mode/3(enum2) -> Bus Creator/4  "PRNDMode_FMWS [enum]"

== system VCMGCM1962020b_v2/Fgnd/Control/Other ==
  Data : Inport
  A/C Compressor : Subsystem  Commented=on
  Brake Vacuum Pump : Subsystem  Commented=on
  Bus Creator : BusCreator  Inputs=8
  Cooling Fan : Subsystem
  Cooling Pumps : Subsystem
  Header : Blocks_lib/Header  width=Portrait  addtext=''
  Heater : Subsystem  Commented=on
  Other : Subsystem
  Park Pawl : Subsystem  Commented=on
  Power Steering Pump : Subsystem  Commented=on
  Ctrl : Outport  VectorParamsAs1DForOutWhenUnconnected=off
  wires:
  Bus Creator/1 -> Ctrl/1  "Other"
  Brake Vacuum Pump/1(Bool) -> Bus Creator/2  "BrkVacuumPump [Bool]"
  Power Steering Pump/1(Ctrl) -> Bus Creator/3
  Cooling Pumps/1(Ctrl) -> Bus Creator/6
  Heater/1(Ctrl) -> Bus Creator/5
  Cooling Fan/1(Bool) -> Bus Creator/7  "CoolFan [Bool]"
  A/C Compressor/1(Ctrl) -> Bus Creator/4
  Other/1(Ctrl) -> Bus Creator/8
  Park Pawl/1(Bool) -> Bus Creator/1  "PrkPawl [Bool]"
  Data/1 -> Park Pawl/1(Data), Power Steering Pump/1(Data), A/C Compressor/1(Data), Heater/1(Data), Cooling Pumps/1(Data), Cooling Fan/1(Data), Other/1(Data), Brake Vacuum Pump/1(Data)

== system VCMGCM1962020b_v2/Fgnd/Control/PDU ==
  Data : Inport
  Bus Creator : BusCreator  Inputs=1
  Bus Selector : BusSelector  Commented=on  OutputSignals=VirtualSensors.Chgr.OffBoard.OffBoardChgrDCChgCntrReq [Bool]
  Header : Blocks_lib/Header  width=Portrait  addtext=''
  High-Voltage Discharge Contactor : Subsystem  Commented=on
  Main  Contactor Cmd : Subsystem  Commented=on  mask{nam='Main', group='Control | PDU'}
      mask prompts: nam "Name"
      mask init:
      | cb = gcb;
      | 
      | % --- Name Line
      | NameLine([cb '/BusCreator'], 'Inport(1)', [nam 'PreChgComplete [Bool]']);
      | NameLine([cb '/BusCreator'], 'Inport(2)', [nam 'PreChgCntr [Bool]']);
      | NameLine([cb '/BusCreator'], 'Inport(3)', [nam 'PosCntr [Bool]']);
      | NameLine([cb '/BusCreator'], 'Inport(4)', [nam 'NegCntr [Bool]']);
      | NameLine([cb '/BusCreator'], 'Outport', [nam 'Cntrs']);
      mask Display: disp(['Pre-Charge and\nContactor Control\n' nam]);
  PDU Contactor Commands : Subsystem  mask{group='Contactor Commands'}
      mask prompts: group "Group Name"
  Zero-Order Hold : ZeroOrderHold  Commented=on  SampleTime=-1
  Ctrl : Outport  VectorParamsAs1DForOutWhenUnconnected=off
  wires:
  Bus Creator/1 -> Ctrl/1  "PDU"
  Bus Selector/1 -> Zero-Order Hold/1  "<OffBoardChgrDCChgCntrReq [Bool]>"
  PDU Contactor Commands/1(Ctrl) -> Bus Creator/1
  Data/1 -> PDU Contactor Commands/1(Data), High-Voltage Discharge Contactor/1(Data), Bus Selector/1

== system VCMGCM1962020b_v2/Fgnd/Diagnostics/Diagnostics ==
  Data : Inport
  A/C Compressor Fault : Subsystem  Commented=on
  "Battery Cell Temperature (avg) High " : Subsystem
  Battery Cell Temperature (max) High : Subsystem
  Battery Cell Voltage (max) High : Subsystem
  Battery Cell Voltage (min) Low : Subsystem
  Battery Current High : Subsystem
  Battery Fault : Subsystem
  CAN Bus Passive : Subsystem
  Charger (off-board) Isolation Fault : Subsystem  Commented=on
  Charger (on-board) Fault : Subsystem
  Contactor SOH Faults : Subsystem  Commented=on
  Contactor X-Checks : Subsystem
  Cooling Pump Fault : Subsystem  Commented=on
  DC/DC Converter Fault : Subsystem
  DC/DC Converter X-Check : Subsystem  Commented=on
  DRVP Voltage High/Low : Subsystem
  Drive Inverter Fault : Subsystem
  Drive Motor Torque X-Check : Subsystem
  E-Stop : Subsystem
  HV Bus Isolation Low : Subsystem
  HV Bus Voltage High : Subsystem
  HVIL X-Check : Subsystem
  Header : Blocks_lib/Header  width=Portrait  addtext=''
  Heater Fault : Subsystem  Commented=on
  Inertia Switch : Subsystem  Commented=on
  MPDM Fuse & Relay Faults : Subsystem  Commented=on
  MPRD Open/Short : Subsystem  Commented=on
  Power Steering Pump Inverter Fault : Subsystem  Commented=on
  XDRP Voltage High/Low : Subsystem
  wires:
  Data/1 -> A/C Compressor Fault/1(Data), Battery Cell Temperature (max) High/1(Data), Battery Cell Voltage (max) High/1(Data), Battery Cell Voltage (min) Low/1(Data), Battery Current High/1(Data), Battery Fault/1(Data), CAN Bus Passive/1(Data), Charger (on-board) Fault/1(Data), Charger (off-board) Isolation Fault/1(Data), "Battery Cell Temperature (avg) High "/1(Data), Contactor SOH Faults/1(Data), Cooling Pump Fault/1(Data), DC/DC Converter Fault/1(Data), DC/DC Converter X-Check/1(Data), DRVP Voltage High/Low/1(Data), Drive Inverter Fault/1(Data), Drive Motor Torque X-Check/1(Data), HV Bus Isolation Low/1(Data), E-Stop/1(Data), Contactor X-Checks/1(Data), HVIL X-Check/1(Data), Heater Fault/1(Data), Inertia Switch/1(Data), MPDM Fuse & Relay Faults/1(Data), MPRD Open/Short/1(Data), Power Steering Pump Inverter Fault/1(Data), XDRP Voltage High/Low/1(Data), HV Bus Voltage High/1(Data)
